simulink model "Controller_Sim"  (R2016a)
settings: Solver=ode1  SolverMode=MultiTasking  StartTime=0.0  StopTime=10  FixedStep=0.0005  RelTol=1e-3
StopFcn:
  | structifySimData
  | ConstructLog_Sim
values from neighbouring files (symbols this model uses):
  ControlParams = input.ControlParams    [Controller.m]    (also in Controller_Yukai.m)
  ControlState = input.ControlState    [Controller.m]    (also in Controller_Yukai.m)
undefined symbols (not defined in the file or in its folder): DiscIntNeverNeededParam, EnablePerturb, EnableStictionModel, FootPoints, gd, get, GroundModel, leg_length, LegHipTorqueLimit, LibWalkingDDA, pL1, pL2, pR1, pR2, ps3Axes, ps3Buttons, ps3Pov, RoughTerrain1, spring_k, spring_zeta, torso_com_offset, Ts, xinit, xLine, yLine, Z
libraries: simulink x5, Friction_Compensator_Lib x2, robotlib x2, vrlib x1
(part 2 of 2)

== matlab function Controller_Sim/Controller/Joystick Parser/xbox_mapping/xbox_cmd_assigner ==
  data: ControlStateIn input; xbox input; ControlStateOut output Bus: ControlState_bus; xboxPrev input
function ControlStateOut = xbox_cmd_assigner(ControlStateIn, xbox, xboxPrev) %#codegen
%% Copyright 2016 - Ross Hartley

ControlStateOut = ControlStateIn;
sampleInterval = 0.0005;

%% Commands 

% Shutdown
if xbox.back == 1
	ControlStateOut.Commands.Shutdown = 1;
end

% Enable
if xbox.start == 1
	ControlStateOut.Commands.EnableTransition = 1;
end

% If rightBumper is pressed, reset state estimator
if (xbox.rightBumper == 1) && (xboxPrev.rightBumper == 0) % Rising edge
	ControlStateOut.Commands.ResetStateEstimator = 1;
else
    ControlStateOut.Commands.ResetStateEstimator = 0;
end

% If leftBumper is pressed, calibrate offsets
if (xbox.leftBumper == 1) && (xboxPrev.leftBumper == 0) % Rising edge
    ControlStateOut.Commands.IntegralControl = ~ControlStateOut.Commands.IntegralControl;
end

% Parse right joystick for time scaling tests
TimeScale = max(min(xbox.rightStickY, 1), -1);
alpha_ts = sampleInterval/(2 + sampleInterval);
ControlStateOut.Commands.TimeScale = ControlStateOut.Commands.TimeScale + alpha_ts*(TimeScale - ControlStateOut.Commands.TimeScale);
% If rightBumper is pressed, pause time
if (xbox.rightBumper == 1) && (xboxPrev.rightBumper == 0) % Rising edge
    ControlStateOut.Commands.PauseTime = ~ControlStateOut.Commands.PauseTime;
end
    
if ControlStateIn.Options.Enable_dy_tgt
    % Parse left joystick data for Y Velocity
    dy_cmd = max(min(xbox.leftStickY, 0.8), -0.8);
    if abs(dy_cmd) < 0.1
        dy_cmd = 0; % Ignore small values
    end
    % Filter target X velocity command
    alpha_dy = sampleInterval/(2 + sampleInterval);
    ControlStateOut.Commands.dy_tgt = ControlStateOut.Commands.dy_tgt + alpha_dy*(dy_cmd - ControlStateOut.Commands.dy_tgt);
end

if ControlStateIn.Options.Enable_dx_tgt
    % Parse right joystick data for X Velocity
    dx_cmd = max(min(xbox.rightStickX, 0.5), -0.5);
    if abs(dx_cmd) < 0.1
        dx_cmd = 0; % Ignore small values
    end
    % Filter target X velocity command
    alpha_dx = sampleInterval/(2 + sampleInterval);
    ControlStateOut.Commands.dx_tgt = ControlStateOut.Commands.dx_tgt + alpha_dx*(dx_cmd - ControlStateOut.Commands.dx_tgt);
end

% Activate Side Stepping
if xbox.X == 1 && ControlStateIn.Options.EnableSideStep
	ControlStateOut.Commands.ActivateSideStepLeft = 1;
else
	ControlStateOut.Commands.ActivateSideStepLeft = 0;
end

% Activate Kicking
if xbox.A == 1 && ControlStateIn.Options.EnableKicking
	ControlStateOut.Commands.ActivateKickingLeft = 1;
else
	ControlStateOut.Commands.ActivateKickingLeft = 0;
end

%% Offsets

% Center of Mass offsets
if (xbox.dUp == 1) && (xboxPrev.dUp == 0) % Rising edge
	ControlStateOut.Offsets.yOffset = ControlStateOut.Offsets.yOffset + 0.001;
end
if (xbox.dDown == 1) && (xboxPrev.dDown == 0) % Rising edge
	ControlStateOut.Offsets.yOffset = ControlStateOut.Offsets.yOffset - 0.001;
end
if (xbox.dRight == 1) && (xboxPrev.dRight == 0) % Rising edge
	ControlStateOut.Offsets.xOffset = ControlStateOut.Offsets.xOffset + 0.001;
end
if (xbox.dLeft == 1) && (xboxPrev.dLeft == 0) % Rising edge
	ControlStateOut.Offsets.xOffset = ControlStateOut.Offsets.xOffset - 0.001;
end


end

== matlab function Controller_Sim/Plant/CheckTerminationCond/MATLAB Function ==
  data: x_e input; terminate_signal output; leg_length input; torso_com_offset input
function terminate_signal  =  CheckTerminationConditions(x_e,leg_length,torso_com_offset)
%#codegen
%
q  = x_e(1:16);
dq = x_e(17:end);

%[pcm p0 p0T pHR p1R p2R p3R p4R pHL p1L p2L p3L p4L] = ATRIAS3D_Primary_PointsHip(q);
[pcm, p0, p0T, pHR, p1R, p2R, p3R, p4R, pHL, p1L, p2L, p3L, p4L] = OriginalLeg_Springs_VariableLeg_COMoffset.ATRIAS3D_Positions_Hip(q,[leg_length;torso_com_offset]);

p_Z = [p4L(3), p4R(3)];

%Terminate if torso top goes below 0.5m or either foot goes above 1 m
if p0T(3)<0.5 %|| max(p_Z) > 1
    terminate_signal = 1;
else    
    terminate_signal = 0;
end

== matlab function Controller_Sim/Controller/Joystick Parser/xbox_parser ==
  data: axis input; xbox output Bus: xbox_bus; buttons input; pov input
function xbox = xbox_parser(axis, buttons, pov)
%#codegen

% axis parsing
xbox.leftStickX = axis(1);
xbox.leftStickY = -axis(2);
xbox.leftTrigger = axis(3);
xbox.rightStickX = axis(4);
xbox.rightStickY = -axis(5);
%xbox.rightTrigger = axis(6);
xbox.rightTrigger = axis(3);

% button parsing
xbox.A = buttons(1);
xbox.B = buttons(2);
xbox.X = buttons(3);
xbox.Y = buttons(4);
xbox.leftBumper = buttons(5);
xbox.rightBumper = buttons(6);
xbox.back = buttons(7);
xbox.start = buttons(8);
xbox.leftStickButton = buttons(9);
xbox.rightStickButton = buttons(10);

% D-pad parsing
switch pov
	case -1
		xbox.dUp = 0;
		xbox.dRight = 0;
		xbox.dDown = 0;
		xbox.dLeft = 0;
		
	case 0
		xbox.dUp = 1;
		xbox.dRight = 0;
		xbox.dDown = 0;
		xbox.dLeft = 0;
		
	case 45
		xbox.dUp = 1;
		xbox.dRight = 1;
		xbox.dDown = 0;
		xbox.dLeft = 0;
		
	case 90
		xbox.dUp = 0;
		xbox.dRight = 1;
		xbox.dDown = 0;
		xbox.dLeft = 0;
		
	case 135
		xbox.dUp = 0;
		xbox.dRight = 1;
		xbox.dDown = 1;
		xbox.dLeft = 0;
		
	case 180
		xbox.dUp = 0;
		xbox.dRight = 0;
		xbox.dDown = 1;
		xbox.dLeft = 0;
		
	case 225
		xbox.dUp = 0;
		xbox.dRight = 0;
		xbox.dDown = 1;
		xbox.dLeft = 1;
	
	case 270
		xbox.dUp = 0;
		xbox.dRight = 0;
		xbox.dDown = 0;
		xbox.dLeft = 1;
		
	case 315
		xbox.dUp = 1;
		xbox.dRight = 0;
		xbox.dDown = 0;
		xbox.dLeft = 1;
		
	otherwise
		xbox.dUp = 0;
		xbox.dRight = 0;
		xbox.dDown = 0;
		xbox.dLeft = 0;
		
end
		
end

== matlab function Controller_Sim/Plant/DennisHarmonicDriveStictionModel/LuGre_Fric_MATLAB/MATLAB Function ==
  data: vel input; p input; Fric output; z input; dz output
function [Fric,dz] = LuGre_Fric_MATLAB(vel,p,z)
%#codegen

% J = p(1);
alpha0 = p(2);
alpha0v2 = p(3);
alpha1 = p(4);
alpha1v2 = p(5);
alpha2 = p(6);
alpha2v2 = p(7);
alpha3 = p(8); 
alpha3v2 = p(9);
v0 = p(10);
v0v2 = p(11);
sigma0 = p(12);
sigma1 = p(13);
fConst = p(14);

x2 = vel*180/pi;
g = (alpha0+alpha1*exp(-(x2/v0).^2))*(x2>=0)+(alpha0v2+alpha1v2*exp(-(x2/v0v2).^2))*(x2<0);
dz = x2-sigma0/g*abs(x2)*z;

Fric = sigma0*z+sigma1*dz+(alpha2*x2)*(x2>=0)+(abs(alpha2v2)*x2)*(x2<0)+(alpha3*x2^2)*(x2>=0)+(-abs(alpha3v2)*x2^2)*(x2<0)+fConst;

== matlab function Controller_Sim/Plant/DennisHarmonicDriveStictionModel/LuGre_Fric_MATLAB1/MATLAB Function ==
  data: vel input; p input; Fric output; z input; dz output
function [Fric,dz] = LuGre_Fric_MATLAB(vel,p,z)
%#codegen

% J = p(1);
alpha0 = p(2);
alpha0v2 = p(3);
alpha1 = p(4);
alpha1v2 = p(5);
alpha2 = p(6);
alpha2v2 = p(7);
alpha3 = p(8); 
alpha3v2 = p(9);
v0 = p(10);
v0v2 = p(11);
sigma0 = p(12);
sigma1 = p(13);
fConst = p(14);

x2 = vel*180/pi;
g = (alpha0+alpha1*exp(-(x2/v0).^2))*(x2>=0)+(alpha0v2+alpha1v2*exp(-(x2/v0v2).^2))*(x2<0);
dz = x2-sigma0/g*abs(x2)*z;

Fric = sigma0*z+sigma1*dz+(alpha2*x2)*(x2>=0)+(abs(alpha2v2)*x2)*(x2<0)+(alpha3*x2^2)*(x2>=0)+(-abs(alpha3v2)*x2^2)*(x2<0)+fConst;

== matlab function Controller_Sim/ROS: Publish Joint States/MATLAB Function - Assign ==
  data: blankMessage input; t input; q input; msg output Bus: SL_Bus_Controller_Sim_v3_trajectory_msgs_JointTrajectory; Ts input
function msg = assign_JointTrajectory(blankMessage, t, q, Ts)
%#codegen

% To set datatype of MSG output:
%  1. Create buses for this model: robotics.ros.createSimulinkBus(gcs)
%  1. Click "Edit Data" in  Toolstrip to open "Ports and Data Manager"
%  2. Select MSG and set datatype to "Bus: SL_Bus_<modelname>_<messageType>"
% See: 
% http://www.mathworks.com/help/simulink/ug/create-structures-in-matlab-function-blocks.html

% blankMessage (nav_msgs/Odometry) consists of
%                Header: [1x1 Header]
%          ChildFrameId: variable-length array of uint8
%  ChildFrameId_SL_Info: struct with fields CurrentLength, ReceivedLength
%                  Pose: [1x1 PoseWithCovariance]
%                 Twist: [1x1 TwistWithCovariance]

% Assign the output message to be the same with input blank message
msg = blankMessage;

%% Modify the nested messages

% Assign Joint Names
strArrayToAssign = {'x', 'y', 'z', 'qz', 'qy', 'qx', 'q1R', 'q2R', 'q3R', ...
    'q1L', 'q2L', 'q3L', 'L1R_to_L4R', 'L2R_to_L3R', 'L1L_to_L4L', 'L2L_to_L3L'};
numStringsInArray = length(strArrayToAssign);
msg.JointNames_SL_Info.CurrentLength = uint32(numStringsInArray);
for idx=1:numStringsInArray
    str = strArrayToAssign{idx};
    strLength = length(str);
    msg.JointNames(idx).Data(1:strLength) = uint8(str);
    msg.JointNames(idx).Data_SL_Info.CurrentLength = uint32(strLength);
end

% Assign Frame Id
str = 'world_gazebo';
strLength = length(str);
msg.Header.FrameId_SL_Info.CurrentLength = uint32(strLength);
msg.Header.FrameId(1:strLength) = uint8(str);


% Assign Joint Positions
msg.Points_SL_Info.CurrentLength = uint32(1); 
msg.Points(1).Positions_SL_Info.CurrentLength = uint32(16);

q_vec = zeros(16,1);
q_vec(1:6) = q(1:6);
q_vec(7:12) = q([11,12,13,14,15,16]); 
q_vec(13) = (q(12) - q(11)); 
q_vec(14) = -(q(12) - q(11)); 
q_vec(15) = (q(15) - q(14)); 
q_vec(16) = -(q(15) - q(14)); 

msg.Points(1).Positions(1:16) = q_vec;
msg.Points(1).TimeFromStart.Nsec = int32(Ts/1e-9);
